simulink model "cruise_control_fechada"  (R2024b)
settings: Solver=VariableStepAuto  StartTime=0.0  StopTime=100.0  FixedStep=1e-3  RelTol=1e-3
values from neighbouring files (symbols this model uses):
  b = f/vinf    [identificarCruiseControl.m]    (also in questao22e.m = b+10; questao23d.m = b+10)
  bc = b    [questao22a.m]    (also in questao22b.m; questao22c.m; questao22d.m; questao22e.m)
  d = 0    [questao22a.m]    (also in questao22b.m; questao22c.m = 300; questao22d.m; questao22e.m)
  Kp = (m/tau - b)    [questao23a.m]    (also in questao23b.m; questao23c.m; questao23d.m; questao23e.m)
  m = b*tau    [identificarCruiseControl.m]    (also in questao22d.m = m+100)
  vr = 30    [questao22a.m]    (also in questao22b.m = 10; questao22c.m = 10; questao22d.m = 10; questao22e.m = 10)
settings Model: Creator=mmaximo  LastModifiedBy=brunn
settings SolverCC: AlgebraicLoopSolver=TrustRegion
settings DebuggingCC: UnconnectedInputMsg=warning  UnconnectedOutputMsg=warning  UnconnectedLineMsg=warning
settings ModelReferenceCC: EnableRefExpFcnMdlSchedulingChecks=on
settings RTWCC: GPUComputeCapability=3.5  DLArmComputeVersion=19.05

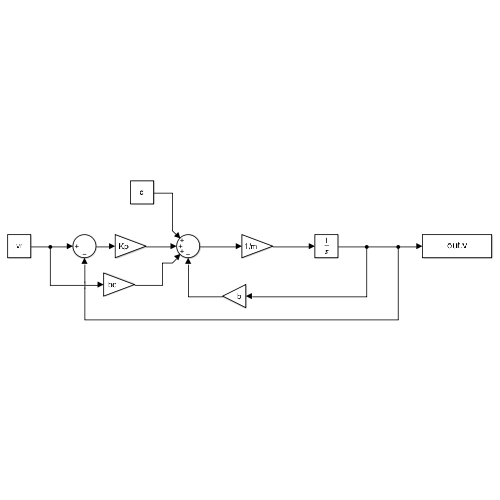
[thumbnail: Simulink's stored preview of the top-level diagram]
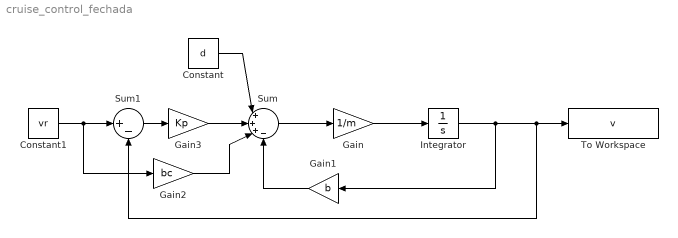
== system cruise_control_fechada ==
  Constant : Constant  Value=d
  Constant1 : Constant  Value=vr
  Gain : Gain  Gain=1/m
  Gain1 : Gain  Gain=b
  Gain2 : Gain  Gain=bc
  Gain3 : Gain  Gain=Kp
  Integrator : Integrator
  Sum : Sum  Inputs=|+++-
  Sum1 : Sum  Inputs=|+-
  To Workspace : ToWorkspace  VariableName=v  SaveFormat=Structure With Time  SampleTime=-1
  wires:
  Gain3/1 -> Sum/2
  Sum/1 -> Gain/1
  Constant/1 -> Sum/1
  Sum1/1 -> Gain3/1
  Gain/1 -> Integrator/1
  Integrator/1 -> Gain1/1, Sum1/2, To Workspace/1
  Gain1/1 -> Sum/4
  Constant1/1 -> Gain2/1, Sum1/1
  Gain2/1 -> Sum/3
